simulink model "BandB"  (Simulink 7.0)
settings: Solver=ode45  StartTime=tstart  StopTime=tstop  RelTol=1e-3
values from neighbouring files (symbols this model uses):
  x0 = p0 * diag([1 1 -1/Bb/G -1/Bb/G]) * [1; 0; -sqrt(-a0); 0]    [BandBinit.m]    (also in EE6283_M9_CE6p2_QuyenHua.m = [10; 10; 10; 10]; EE6283_M9_CME6p4_QuyenHua.m = [10; 10; 10; 10]; EE6283_M9_NE6p3_QuyenHua.m = [10; 10]; InvPendInit.m = [0 0 0 0])
settings Model: Creator=Doug  LastModifiedBy=Doug
settings DataIOCC: LimitDataPoints=off  SaveOutput=off  SignalLogging=off  SaveTime=off
settings DebuggingCC: SolverPrmCheckMsg=none

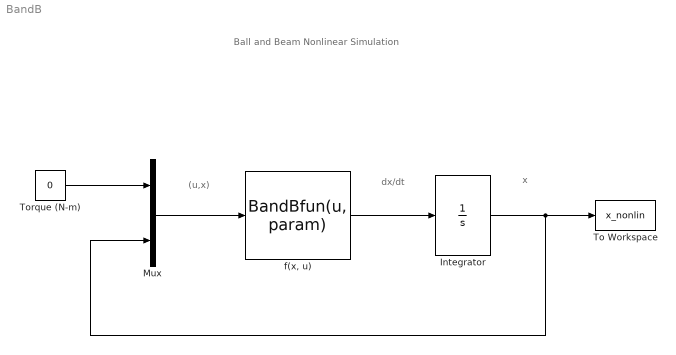
== system BandB ==
  note: Ball and Beam Nonlinear Simulation
  note: dx/dt
  note: x
  note: (u,x)
  Integrator : Integrator  InitialCondition=x0
  Mux : Mux  Inputs=[1 4]
  To Workspace : ToWorkspace  VariableName=x_nonlin  SampleTime=-1  SaveFormat=Structure With Time
  Torque (N-m) : Constant  Value=0  OutDataType=sfix(16)  OutScaling=2^0
  "f(x, u)" : MATLABFcn  MATLABFcn=BandBfun(u, param)
  wires:
  "f(x, u)"/1 -> Integrator/1
  Mux/1 -> "f(x, u)"/1
  Torque (N-m)/1 -> Mux/1
  Integrator/1 -> Mux/2, To Workspace/1
